simulink model "simulazione_007_s"  (R2016b)
settings: Solver=ode4  StartTime=0.0  StopTime=t_sim  FixedStep=step  RelTol=1e-3
undefined symbols (not defined in the file or in its folder): motion_time, movement_lower_limit, movement_upper_limit, p_init, q_init, theta, velocity_lower_limit, velocity_upper_limit
settings Model: Creator=IBM  LastModifiedBy=IBM

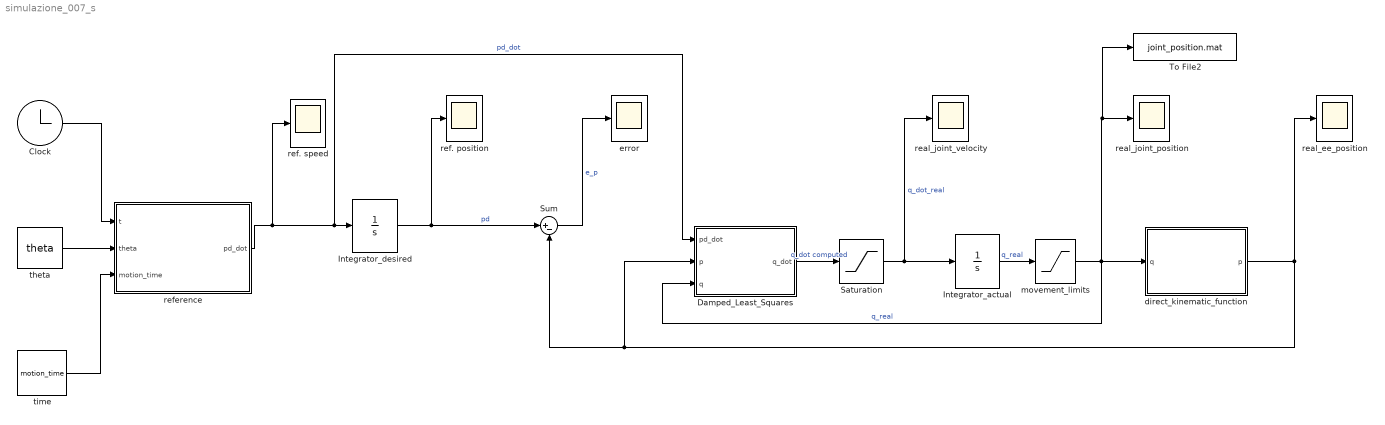
== system simulazione_007_s ==
  Clock : Clock
  Damped_Least_Squares : MATLAB Function  TreatAsAtomicUnit=on
  Integrator_actual : Integrator  InitialCondition=q_init
  Integrator_desired : Integrator  InitialCondition=p_init
  Saturation : Saturate  UpperLimit=velocity_upper_limit  LowerLimit=velocity_lower_limit
  Sum : Sum  Inputs=|+-
  To File2 : ToFile  Filename=joint_position.mat  MatrixName=q
  direct_kinematic_function : MATLAB Function  TreatAsAtomicUnit=on
  error : Scope
  movement_limits : Saturate  UpperLimit=movement_upper_limit  LowerLimit=movement_lower_limit
  real_ee_position : Scope
  real_joint_position : Scope
  real_joint_velocity : Scope
  ref. position : Scope
  ref. speed : Scope
  reference : MATLAB Function  TreatAsAtomicUnit=on
  theta : Constant  Value=theta
  time : Constant  Value=motion_time
  wires:
  Clock/1 -> reference/1(t)
  Integrator_desired/1 -> ref. position/1, Sum/1  "pd"
  Sum/1 -> error/1  "e_p"
  Integrator_actual/1 -> movement_limits/1  "q_real"
  direct_kinematic_function/1(p) -> real_ee_position/1, Damped_Least_Squares/2(p), Sum/2
  theta/1 -> reference/2(theta)
  reference/1(pd_dot) -> ref. speed/1, Damped_Least_Squares/1(pd_dot), Integrator_desired/1  "pd_dot"
  time/1 -> reference/3(motion_time)
  movement_limits/1 -> Damped_Least_Squares/3(q), To File2/1, real_joint_position/1, direct_kinematic_function/1(q)  "q_real"
  Damped_Least_Squares/1(q_dot) -> Saturation/1  "q_dot computed"
  Saturation/1 -> real_joint_velocity/1, Integrator_actual/1  "q_dot_real"

== matlab function simulazione_007_s/Damped_Least_Squares ==
  data: pd_dot input; p input; q_dot output; q input
function q_dot = dls(pd_dot, p, q)
        
    Jg = geometric_jacobian(q);
    Ja = analytic_jacobian(Jg, p);
    
    s = svd(Ja);
    sigma_th = 1/pi;
    sigma = s(6);
    lambda_max = 0.001;
    
    if sigma >= sigma_th 
        lambda = 0; 
    else
        lambda = lambda_max - lambda_max * sigma / sigma_th;
    end
    
    q_dot = transpose(Ja) * inv(Ja * transpose(Ja) + lambda * eye(6)) * pd_dot;
    
end

== matlab function simulazione_007_s/reference ==
  data: t input; theta input; pd_dot output; motion_time input
function pd_dot = reference(t, theta, motion_time)

    pd_dot = rotational_reference(t, theta, motion_time);
    
end

== matlab function simulazione_007_s/direct_kinematic_function ==
  data: q input; p output
function p = dkf(q)

    p = direct_kinematic(q);
